simulink model "Send_IMU_value"  (R2016b)
settings: Solver=FixedStepDiscrete  StartTime=0.0  StopTime=10.0  FixedStep=0.002  RelTol=1e-3
PreLoadFcn:
  | waijung.modelPreload; % Required for working with Waijung Blockset. Do not remove.
InitFcn:
  | cubeparameters
values from neighbouring files (symbols this model uses):
  C = [1 0 0 0 0 0 0 1 0 0 0 0 ... (36 elements, 6x6)]    [K_lqr_3D.mat]
undefined symbols (not defined in the file or in its folder): a_x, a_y, a_z, in1, in2, in3, in4, in5, in6, Link, LQFP100, MadgwickAHRSupdateIMU3, out1, out2, out3, out4, q_0, q_1, q_2, q_3, ST, STM32F407VG, STM32F4DISCOVERY, w_x, w_y, w_z
libraries: simulink x8, waijung_customcode x1, stm32f4_device_config_lib x1, BC_USB x1
(part 2 of 2)

== matlab function Send_IMU_value/SPI3 get Data4/Take away Sensor fail reading2 ==
  data: y output; new input; old input
function y = fcn(new, old)
%#codegen
if(new > -257 && new < -200)
   y = old;
else
    y = new;
end
